simulink model "admittance_controller_quat"  (R2021b)
settings: Solver=FixedStepAuto  StartTime=0.0  StopTime=10.0  RelTol=1e-3
undefined symbols (not defined in the file): dw_d, h_0e, q_d, T_d, w_d
settings Model: Creator=Martin  LastModifiedBy=Martin

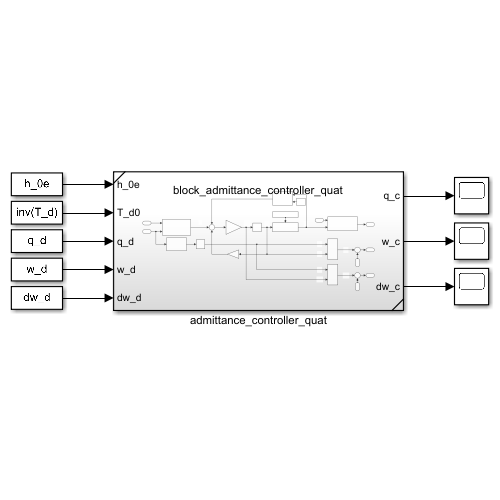
[thumbnail: Simulink's stored preview of the top-level diagram]
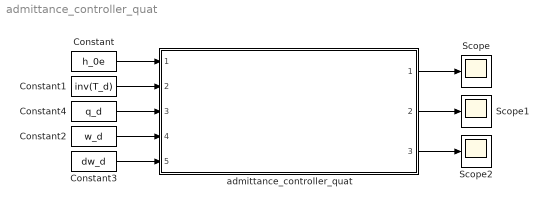
== system admittance_controller_quat ==
  Constant : Constant  Value=h_0e  VectorParams1D=off
  Constant1 : Constant  Value=inv(T_d)
  Constant2 : Constant  Value=w_d  VectorParams1D=off
  Constant3 : Constant  Value=dw_d  VectorParams1D=off
  Constant4 : Constant  Value=q_d  VectorParams1D=off
  Scope : Scope
  Scope1 : Scope
  Scope2 : Scope
  admittance_controller_quat : Subsystem  ReferencedSubsystem=block_admittance_controller_quat
  wires:
  Constant/1 -> admittance_controller_quat/1
  Constant2/1 -> admittance_controller_quat/4
  Constant3/1 -> admittance_controller_quat/5
  admittance_controller_quat/1 -> Scope/1
  admittance_controller_quat/2 -> Scope1/1
  admittance_controller_quat/3 -> Scope2/1
  Constant4/1 -> admittance_controller_quat/3
  Constant1/1 -> admittance_controller_quat/2
